simulink model "prob3"  (R2020b)
settings: Solver=VariableStepAuto  StartTime=0.0  StopTime=10.0  RelTol=1e-3
settings Model: Creator=Nitin  LastModifiedBy=Nitin

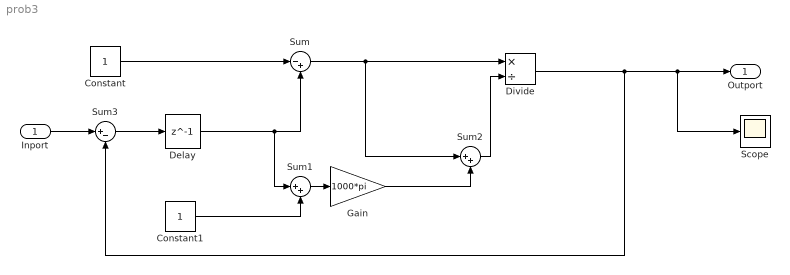
== system prob3 ==
  Inport : Inport
  Constant : Constant
  Constant1 : Constant
  Delay : Delay  DelayLength=1
  Divide : Product  Inputs=*/
  Gain : Gain  Gain=1000*pi
  Scope : Scope
  Sum : Sum  Inputs=|-+
  Sum1 : Sum  Inputs=|++
  Sum2 : Sum  Inputs=|++
  Sum3 : Sum  Inputs=|+-
  Outport : Outport
  wires:
  Sum1/1 -> Gain/1
  Sum/1 -> Divide/1, Sum2/1
  Gain/1 -> Sum2/2
  Sum2/1 -> Divide/2
  Delay/1 -> Sum1/1, Sum/2
  Divide/1 -> Sum3/2, Scope/1, Outport/1
  Constant1/1 -> Sum1/2
  Constant/1 -> Sum/1
  Sum3/1 -> Delay/1
  Inport/1 -> Sum3/1
